simulink model "selector5"  (R2017b)
settings: Solver=FixedStepDiscrete  StartTime=0.0  StopTime=10.0  FixedStep=0.200000  RelTol=1e-3  EnableMultiTasking=on
model workspace (MAT data in the model file):
  already_pp = 0
settings Model: Creator=hbourbou  LastModifiedBy=hbourbou
settings DataIOCC: LimitDataPoints=on  SaveFormat=Structure
settings OptimizationCC: LifeSpan=inf
settings DebuggingCC: AlgebraicLoopMsg=error  ArtificialAlgebraicLoopMsg=error  SFUnexpectedBacktrackingDiag=warning  SFNoUnconditionalDefaultTransitionDiag=warning  SFExecutionAtInitializationDiag=none
settings HardwareCC: ProdBitPerPointer=32  ProdBitPerSizeT=32  ProdBitPerPtrDiffT=32  ProdLargestAtomicFloat=None  ProdIntDivRoundTo=Undefined  ProdEndianess=Unspecified  ProdWordSize=32  ProdHWDeviceType=32-bit Generic
settings ModelReferenceCC: PropagateSignalLabelsOutOfModel=off
settings CodeAppCC: StateflowObjectComments=on
settings GRTTargetCC: TargetLangStandard=C89/C90 (ANSI)  GeneratePreprocessorConditionals=Disable all
settings ConfigComp: CovMetricSettings=dw  CovHtmlReporting=on  CovSaveCumulativeToWorkspaceVar=on  CovSaveSingleToWorkspaceVar=on  CovExternalEMLEnable=off

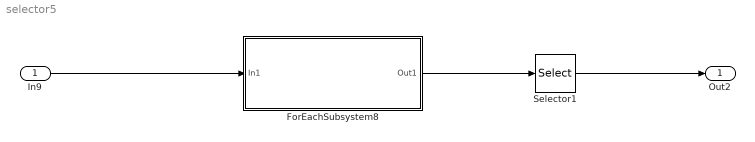
== system selector5 ==
  In9 : Inport  OutDataTypeStr=double  PortDimensions=[3 2 4]
  ForEachSubsystem8 : Subsystem  TreatAsAtomicUnit=on
  Selector1 : Selector  NumberOfDimensions=3  InputPortWidth=3  IndexOptions=Select all,Select all,Index vector (dialog)  Indices=[1 3],1,1  OutputSizes=1,1,1
  Out2 : Outport
  wires:
  In9/1 -> ForEachSubsystem8/1(In1)
  ForEachSubsystem8/1(Out1) -> Selector1/1
  Selector1/1 -> Out2/1

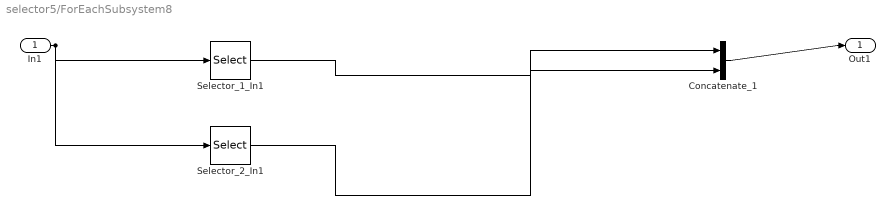
== system selector5/ForEachSubsystem8 ==
  In1 : Inport  OutDataTypeStr=double  PortDimensions=[3 2 4]
  Concatenate_1 : Concatenate  Mode=Multidimensional array
  Selector_1_In1 : Selector  NumberOfDimensions=3  IndexOptions=Select all,Select all,Index vector (dialog)  Indices=,,[1 2]  OutputSizes=1
  Selector_2_In1 : Selector  NumberOfDimensions=3  IndexOptions=Select all,Select all,Index vector (dialog)  Indices=,,[3 4]  OutputSizes=1
  Out1 : Outport
  wires:
  Concatenate_1/1 -> Out1/1
  Selector_2_In1/1 -> Concatenate_1/2
  Selector_1_In1/1 -> Concatenate_1/1
  In1/1 -> Selector_2_In1/1, Selector_1_In1/1
